simulink library "paullib"  (R2023b)
settings: Solver=VariableStepAuto  StartTime=0.0  StopTime=10.0  RelTol=1e-3
libraries: dspxfrm3 x1, dspmtrx3 x1
settings Model: Creator=pbroo  LastModifiedBy=pbroo

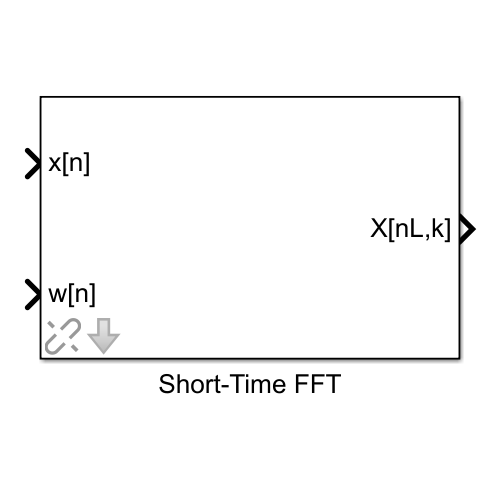
[thumbnail: Simulink's stored preview of the top-level diagram]
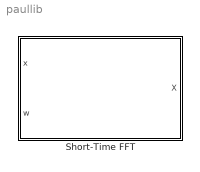
== system paullib ==
  Short-Time FFT : Subsystem  AncestorBlock=dspxfrm3/Short-Time FFT  mask(Short-Time FFT){W=512, OvLap=384, M=1024}
      mask prompts: W "dsp:DSPTransformsBlockDialog:WindowLength_MP"; OvLap "dsp:DSPTransformsBlockDialog:OverlapBetweenWindows_MP"; M "dsp:DSPTransformsBlockDialog:FFTLength_MP"
      mask help: dsp:DSPTransformsBlockDialog:STFT_MaskDesc
      mask init:
      | if W == 1
      |     error('spblockset:ShortTimeFFT:winLenOne', ...
      |           'The analysis window length must be greater than 1');
      | end
      | 
      | L = W-OvLap;
      mask Help: eval('blocksethelp');
      mask DialogControl W Prompt: Analysis window length:
      mask DialogControl OvLap Prompt: Overlap between consecutive windows (in samples):
      mask DialogControl M Prompt: FFT length:
      mask Display:
      | port_label('input',1,'x[n]')
      | port_label('input',2,'w[n]')
      | port_label('output',1,'X[nL,k]')

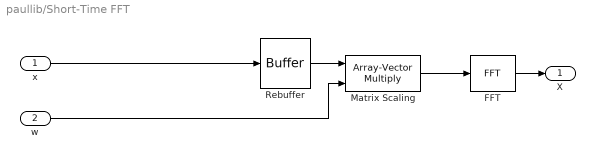
== system paullib/Short-Time FFT ==
  x : Inport
  w : Inport  Port=2
  FFT : dspxfrm3/FFT  FFTImplementation=Auto  CompMethod=Table lookup  TableOpt=NEW  TableOptActive=Speed  BitRevOrder=off  Normalize=off  InheritFFTLength=off  FFTLength=M  WrapInput=on  roundingMode=Floor  overflowMode=off  firstCoeffDataTypeStr=Inherit: Same word length as input  firstCoeffLastDataTypeStr=Inherit: Same word length as input  outputMin=[]  outputMax=[]
  Matrix Scaling : dspmtrx3/Array-Vector Multiply  mode=Mute  saveAsFlag=0  Dimension=1  V_Source=Input port  V_VectFromMask=[0.5 0.25]  roundingMode=Floor  overflowMode=off  firstCoeffSignedness=Auto  firstCoeffDataTypeStr=Inherit: Same word length as input  firstCoeffMin=[]  firstCoeffMax=[]  firstCoeffLastDataTypeStr=Inherit: Same word length as input  prodOutputSignedness=Auto  accumSignedness=Auto  outputSignedness=Auto  outputMin=[]  outputMax=[]
  Rebuffer : Buffer  N=W  V=W-L  OutputFrames=off
  X : Outport  VectorParamsAs1DForOutWhenUnconnected=off
  wires:
  FFT/1 -> X/1
  w/1 -> Matrix Scaling/2
  x/1 -> Rebuffer/1
  Rebuffer/1 -> Matrix Scaling/1
  Matrix Scaling/1 -> FFT/1
